simulink model "ksp_zad14"  (Simulink 2.20)
settings: Solver=ode45  StartTime=0.0  StopTime=90.0  RelTol=1e-3  AbsTol=1e-6
settings Model: ConsistencyChecking=off  RTWPlaceOutputsASAP=off

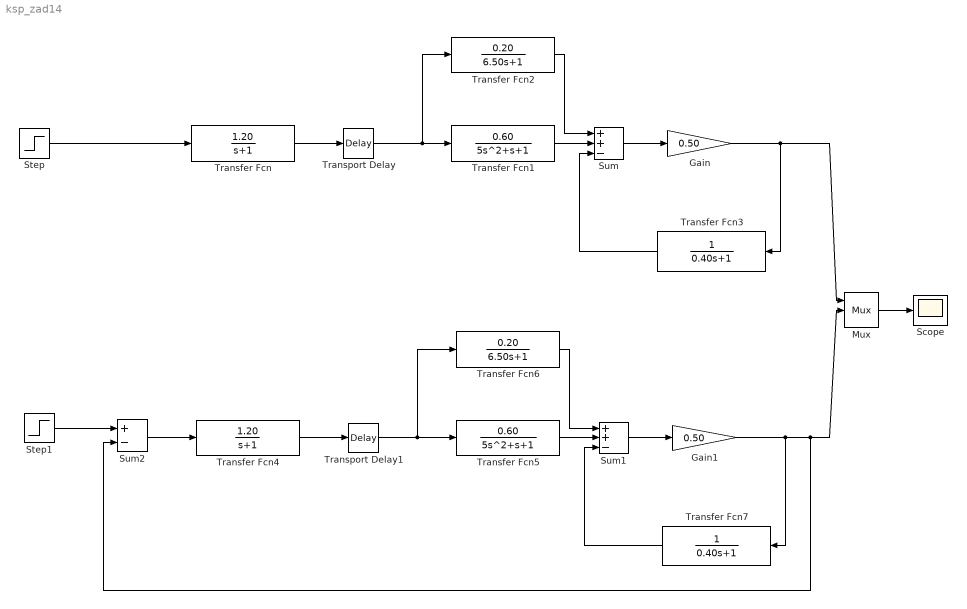
== system ksp_zad14 ==
  Gain : Gain  Gain=0.50
  Gain1 : Gain  Gain=0.50
  Mux : Mux  Inputs=3
  Scope : Scope
      settings: TickLabels=on  TimeRange=90  YMin=-0.05  YMax=0.5  SaveToWorkspace=off  SaveName=ScopeData
  Step : Step  Time=0  Before=0  After=1
  Step1 : Step  Time=0  Before=0  After=1
  Sum : Sum  Inputs=++-
  Sum1 : Sum  Inputs=++-
  Sum2 : Sum  Inputs=+-
  Transfer Fcn : TransferFcn  Numerator=[1.20]  Denominator=[1 1]
  Transfer Fcn1 : TransferFcn  Numerator=[0.60]  Denominator=[5 1 1]
  Transfer Fcn2 : TransferFcn  Numerator=[0.20]  Denominator=[6.50 1]
  Transfer Fcn3 : TransferFcn  Orientation=left  Numerator=[1]  Denominator=[0.40 1]
  Transfer Fcn4 : TransferFcn  Numerator=[1.20]  Denominator=[1 1]
  Transfer Fcn5 : TransferFcn  Numerator=[0.60]  Denominator=[5 1 1]
  Transfer Fcn6 : TransferFcn  Numerator=[0.20]  Denominator=[6.50 1]
  Transfer Fcn7 : TransferFcn  Orientation=left  Numerator=[1]  Denominator=[0.40 1]
  Transport Delay : TransportDelay  DelayTime=2.40  InitialInput=0  BufferSize=1024
  Transport Delay1 : TransportDelay  DelayTime=2.40  InitialInput=0  BufferSize=1024
  wires:
  Transfer Fcn1/1 -> Sum/2
  Transfer Fcn2/1 -> Sum/1
  Sum/1 -> Gain/1
  Transfer Fcn3/1 -> Sum/3
  Transfer Fcn/1 -> Transport Delay/1
  Transport Delay/1 -> Transfer Fcn1/1, Transfer Fcn2/1
  Step/1 -> Transfer Fcn/1
  Mux/1 -> Scope/1
  Gain/1 -> Transfer Fcn3/1, Mux/1
  Sum1/1 -> Gain1/1
  Transfer Fcn7/1 -> Sum1/3
  Transfer Fcn4/1 -> Transport Delay1/1
  Gain1/1 -> Transfer Fcn7/1, Sum2/2, Mux/2
  Transport Delay1/1 -> Transfer Fcn5/1, Transfer Fcn6/1
  Transfer Fcn6/1 -> Sum1/1
  Sum2/1 -> Transfer Fcn4/1
  Step1/1 -> Sum2/1
  Transfer Fcn5/1 -> Sum1/2
